simulink model "ClassicalControlSystems"  (R2021a)
settings: Solver=VariableStepAuto  StartTime=0.0  StopTime=50  MaxStep=10e-3  RelTol=1e-3
libraries: slctrlblks x1, pid_lib x1
settings Model: Creator=User  LastModifiedBy=User

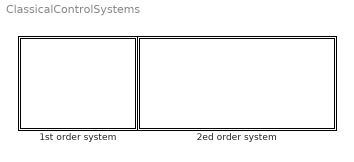
== system ClassicalControlSystems ==
  1st order system : Subsystem
  2ed order system : Subsystem

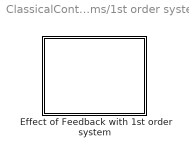
== system ClassicalControlSystems/1st order system ==
  Effect of Feedback with 1st order system : Subsystem

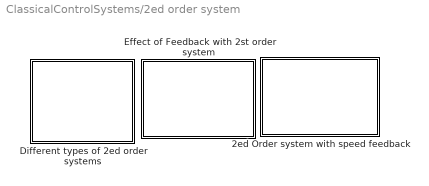
== system ClassicalControlSystems/2ed order system ==
  2ed Order system with speed feedback : Subsystem
  Different types of 2ed order systems : Subsystem
  Effect of Feedback with 2st order system : Subsystem

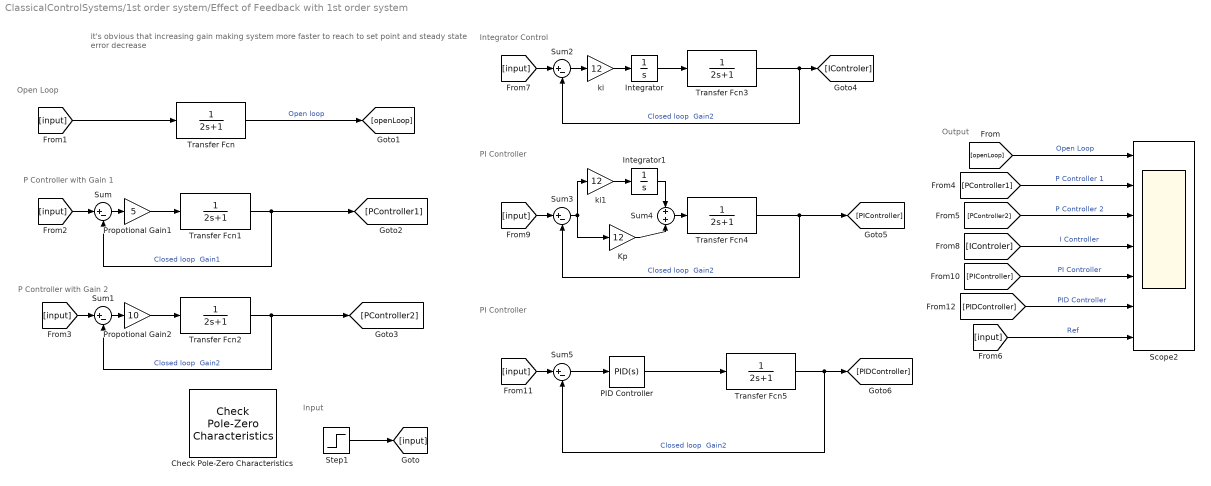
== system ClassicalControlSystems/1st order system/Effect of Feedback with 1st order system ==
  note: Output
  note: Integrator Control
  note: P Controller with Gain 2
  note: P Controller with Gain 1
  note: Open Loop
  note: Input
  note: it's obvious that increasing gain making system more faster to reach to set point and steady state error decrease
  note: PI Controller
  note: PI Controller
  Check Pole-Zero Characteristics : slctrlblks/Model Verification/Check Pole-Zero Characteristics  InstantiateOnLoad=on  SaveOperatingPoints=off  LinearizationIOs={}  LinearizeAt=SnapshotTimes  SnapshotTimes=[0]  TriggerType=rising  SampleTime=auto  RateConversionMethod=zoh  PreWarpFreq=10  UseExactDelayModel=off  UseFullBlockNameLabels=off  UseBusSignalLabels=off  enabled=on  stopWhenAssertionFail=off  export=off  ViewDlgPos=[]  LaunchViewOnOpen=off  OpenViewOnLoad=off  FrequencyUnits=rad/s  MagnitudeUnits=dB  PhaseUnits=deg  TimeUnits=seconds  EnableSettlingTime=on  SettlingTime=1  EnablePercentOvershoot=on  PercentOvershoot=10  EnableDampingRatio=off  DampingRatio=[]  EnableNaturalFrequency=off  NaturalFrequencyBound=>=  NaturalFrequency=[]
      settings: SourceProductBaseCode=SD  SaveToWorkspace=off  SaveName=sys
  Integrator : Integrator
  Integrator1 : Integrator
  Kp : Gain  Gain=12
  PID Controller : pid_lib/PID Controller  Controller=PID  Form=Parallel  TimeDomain=Continuous-time  UseExternalTs=off  SampleTime=-1  IntegratorMethod=Forward Euler  FilterMethod=Forward Euler  ControllerParametersSource=internal  P=2511.45586336671  I=577566.277854476  D=0.262938326903842  UseFilter=on  N=7020.21600074244  TunerSelectOption=Transfer Function Based (PID Tuner App)  InitialConditionSource=internal  InitialConditionForIntegrator=0  InitialConditionForFilter=0  DifferentiatorICPrevScaledInput=0  ExternalReset=none  TrackingMode=off  Kt=1  LimitOutput=off  SatLimitsSource=internal  UpperSaturationLimit=inf  LowerSaturationLimit=-inf  LinearizeAsGain=on  AntiWindupMode=none  Kb=1  POutMin=[]  POutMax=[]  IOutMin=[]  IOutMax=[]  DOutMin=[]  DOutMax=[]  NOutMin=[]  NOutMax=[]  SumOutMin=[]  SumOutMax=[]  SaturationOutMin=[]  SaturationOutMax=[]  PParamMin=[]  PParamMax=[]  IParamMin=[]  IParamMax=[]  DParamMin=[]  DParamMax=[]  NParamMin=[]  NParamMax=[]  KbParamMin=[]  KbParamMax=[]  KtParamMin=[]  KtParamMax=[]  KbOutMin=[]  KbOutMax=[]  KtOutMin=[]  KtOutMax=[]  IntegratorOutMin=[]  IntegratorOutMax=[]  FilterOutMin=[]  FilterOutMax=[]  SumI1OutMin=[]  SumI1OutMax=[]  SumI2OutMin=[]  SumI2OutMax=[]  SumI3OutMin=[]  SumI3OutMax=[]  SumI4OutMin=[]  SumI4OutMax=[]  SumDOutMin=[]  SumDOutMax=[]  DifferentiatorOutMin=[]  DifferentiatorOutMax=[]  FilterDiffOutCoefMin=[]  FilterDiffOutCoefMax=[]  ReciprocalOutMin=[]  ReciprocalOutMax=[]  SumDenOutMin=[]  SumDenOutMax=[]  SumNumOutMin=[]  SumNumOutMax=[]  DivideOutMin=[]  DivideOutMax=[]  UdiffTsProdOutMin=[]  UdiffTsProdOutMax=[]  NTsProdOutMin=[]  NTsProdOutMax=[]  UintegralTsProdOutMin=[]  UintegralTsProdOutMax=[]  UngainTsProdOutMin=[]  UngainTsProdOutMax=[]  IntegratorContinuousStateAttributes=''  IntegratorStateMustResolveToSignalObject=off  IntegratorRTWStateStorageClass=Auto  FilterContinuousStateAttributes=''  FilterStateMustResolveToSignalObject=off  FilterRTWStateStorageClass=Auto  ParallelPVariant=InternalParameters  IdealPVariant=Disabled  IVariant=InternalParameters  DVariant=InternalParameters  IntegratorVariant=Continuous  SatVariant=Disabled  AWVariant=Passthrough  PCopyVariant=Disabled  TRVariant=Disabled  FdbkBlocksVariant=Forward  IdealPFdbkVariant=Disabled  SatFdbkVariant=Disabled  DerivativeFilterVariant=ContFilter  NVariant=InternalParameters  NCopyVariant=Disabled  FilterICVariant=InternalICsFilter  IntegratorICVariant=InternalICs  ExternalResetVariant=Disabled  TRSumVariant=Passthrough  SumFdbkVariant=Disabled  SumVariant=Sum_PID  TsampFilterVariant=InternalTs  TsampNgainVariant=Passthrough  TsampIntegralVariant=Passthrough  ExternalSaturationOutDataTypeStr=Inherit: Same as second input
  Propotional Gain1 : Gain  Gain=5
  Propotional Gain2 : Gain  Gain=10
  Scope2 : Scope  NumInputPorts=7
  Step1 : Step  SampleTime=0
  Sum{,1..3,5} (5 alike) : Sum  Inputs=|+-
  Sum4 : Sum  Inputs=+|+
  Transfer Fcn{,1..5} (6 alike) : TransferFcn  Denominator=[2 1]
  ki : Gain  Gain=12
  ki1 : Gain  Gain=12
  wires:
  Propotional Gain1/1 -> Transfer Fcn1/1
  Step1/1 -> [input]
  Sum/1 -> Propotional Gain1/1
  Transfer Fcn1/1 -> [PController1], Sum/2  "Closed loop  Gain1"
  Transfer Fcn/1 -> [openLoop]  "Open loop"
  [input] -> Transfer Fcn/1
  [input] -> Sum/1
  [input] -> Sum1/1
  Transfer Fcn2/1 -> Sum1/2, [PController2]  "Closed loop  Gain2"
  Sum1/1 -> Propotional Gain2/1
  Propotional Gain2/1 -> Transfer Fcn2/1
  [openLoop] -> Scope2/1  "Open Loop"
  [PController1] -> Scope2/2  "P Controller 1"
  [PController2] -> Scope2/3  "P Controller 2"
  ki/1 -> Integrator/1
  Sum2/1 -> ki/1
  Transfer Fcn3/1 -> [IControler], Sum2/2  "Closed loop  Gain2"
  [input] -> Sum2/1
  Integrator/1 -> Transfer Fcn3/1
  [input] -> Scope2/7  "Ref"
  [IControler] -> Scope2/4  "I Controller"
  Integrator1/1 -> Sum4/1
  [input] -> Sum3/1
  Transfer Fcn4/1 -> Sum3/2, [PIController]  "Closed loop  Gain2"
  Sum3/1 -> Kp/1, ki1/1
  ki1/1 -> Integrator1/1
  Sum4/1 -> Transfer Fcn4/1
  Kp/1 -> Sum4/2
  [PIController] -> Scope2/5  "PI Controller"
  PID Controller/1 -> Transfer Fcn5/1
  Transfer Fcn5/1 -> [PIDController], Sum5/2  "Closed loop  Gain2"
  [input] -> Sum5/1
  [PIDController] -> Scope2/6  "PID Controller"
  Sum5/1 -> PID Controller/1

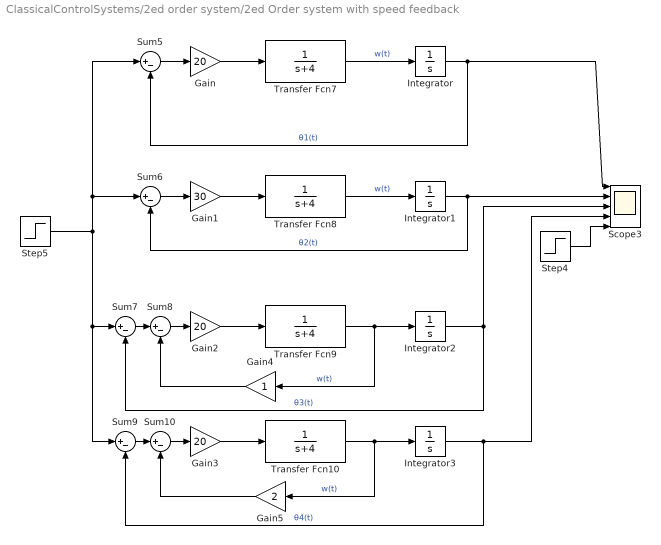
== system ClassicalControlSystems/2ed order system/2ed Order system with speed feedback ==
  Gain : Gain  Gain=20
  Gain1 : Gain  Gain=30
  Gain2 : Gain  Gain=20
  Gain3 : Gain  Gain=20
  Gain4 : Gain
  Gain5 : Gain  Gain=2
  Integrator{,1..3} (4 alike) : Integrator
  Scope3 : Scope  NumInputPorts=5
  Step4 : Step  SampleTime=0
  Step5 : Step  SampleTime=0
  Sum{5..10} (6 alike) : Sum  Inputs=|+-
  Transfer Fcn{7..10} (4 alike) : TransferFcn  Denominator=[1 4]
  wires:
  Step4/1 -> Scope3/5
  Integrator2/1 -> Scope3/3, Sum7/2  "θ3(t)"
  Integrator/1 -> Sum5/2, Scope3/1  "θ1(t)"
  Transfer Fcn10/1 -> Integrator3/1, Gain5/1  "w(t)"
  Transfer Fcn7/1 -> Integrator/1  "w(t)"
  Sum6/1 -> Gain1/1
  Integrator1/1 -> Sum6/2, Scope3/2  "θ2(t)"
  Sum5/1 -> Gain/1
  Step5/1 -> Sum6/1, Sum5/1, Sum7/1, Sum9/1
  Gain1/1 -> Transfer Fcn8/1
  Transfer Fcn8/1 -> Integrator1/1  "w(t)"
  Gain/1 -> Transfer Fcn7/1
  Transfer Fcn9/1 -> Gain4/1, Integrator2/1  "w(t)"
  Gain4/1 -> Sum8/2
  Gain2/1 -> Transfer Fcn9/1
  Sum7/1 -> Sum8/1
  Gain5/1 -> Sum10/2
  Integrator3/1 -> Scope3/4, Sum9/2  "θ4(t)"
  Sum10/1 -> Gain3/1
  Sum8/1 -> Gain2/1
  Gain3/1 -> Transfer Fcn10/1
  Sum9/1 -> Sum10/1

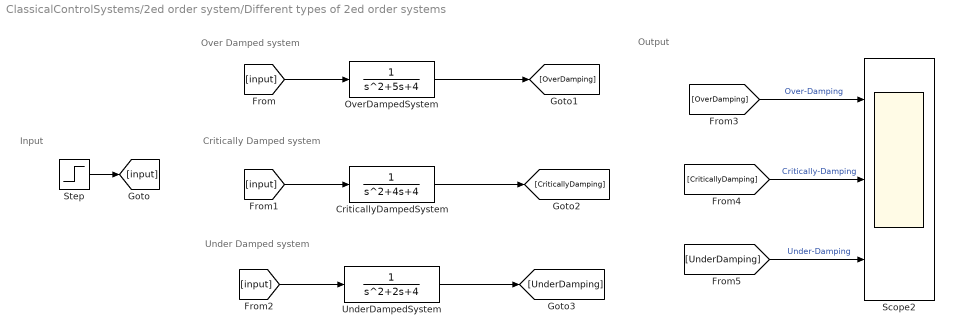
== system ClassicalControlSystems/2ed order system/Different types of 2ed order systems ==
  note: Under Damped system
  note: Critically Damped system
  note: Over Damped system
  note: Input
  note: Output
  CriticallyDampedSystem : TransferFcn  Denominator=[1 4 4]
  OverDampedSystem : TransferFcn  Denominator=[1 5 4]
  Scope2 : Scope  NumInputPorts=3
  Step : Step  SampleTime=0
  UnderDampedSystem : TransferFcn  Denominator=[1 2 4]
  wires:
  CriticallyDampedSystem/1 -> [CriticallyDamping]
  UnderDampedSystem/1 -> [UnderDamping]
  OverDampedSystem/1 -> [OverDamping]
  Step/1 -> [input]
  [input] -> OverDampedSystem/1
  [input] -> CriticallyDampedSystem/1
  [input] -> UnderDampedSystem/1
  [OverDamping] -> Scope2/1  "Over-Damping"
  [CriticallyDamping] -> Scope2/2  "Critically-Damping"
  [UnderDamping] -> Scope2/3  "Under-Damping"

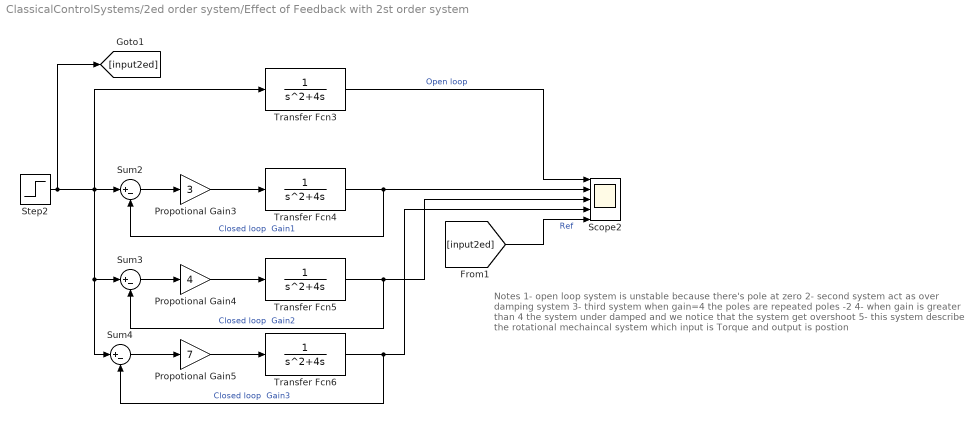
== system ClassicalControlSystems/2ed order system/Effect of Feedback with 2st order system ==
  note: Notes
      | 1- open loop system is unstable because there's pole at zero
      | 2- second system act as over damping system
      | 3- third system when gain=4 the poles are repeated poles -2
      | 4- when gain is greater than 4 the system under damped and we notice that the system get overshoot
      | 5- this system describe the rotational mechaincal system which input is Torque and output is postion
  Propotional Gain3 : Gain  Gain=3
  Propotional Gain4 : Gain  Gain=4
  Propotional Gain5 : Gain  Gain=7
  Scope2 : Scope  NumInputPorts=5
  Step2 : Step  SampleTime=0
  Sum2 : Sum  Inputs=|+-
  Sum3 : Sum  Inputs=|+-
  Sum4 : Sum  Inputs=|+-
  Transfer Fcn{3..6} (4 alike) : TransferFcn  Denominator=[1 4 0]
  wires:
  Sum4/1 -> Propotional Gain5/1
  Transfer Fcn3/1 -> Scope2/1  "Open loop"
  Transfer Fcn6/1 -> Scope2/4, Sum4/2  "Closed loop  Gain3"
  Sum2/1 -> Propotional Gain3/1
  Propotional Gain5/1 -> Transfer Fcn6/1
  Sum3/1 -> Propotional Gain4/1
  Transfer Fcn4/1 -> Scope2/2, Sum2/2  "Closed loop  Gain1"
  Propotional Gain3/1 -> Transfer Fcn4/1
  Propotional Gain4/1 -> Transfer Fcn5/1
  Step2/1 -> Sum2/1, Sum4/1, Sum3/1, Transfer Fcn3/1, [input2ed]
  Transfer Fcn5/1 -> Scope2/3, Sum3/2  "Closed loop  Gain2"
  [input2ed] -> Scope2/5  "Ref"
